simulink model "Model_simulink"  (R2015a)
settings: Solver=ode45  SolverMode=SingleTasking  StartTime=0.0  StopTime=20  RelTol=1e-3
values from neighbouring files (symbols this model uses):
  In = 130.7    [Skrypt_do_schematu.m]
  J = Js+Jmr    (= 5.82)    [Skrypt_do_schematu.m]
  Kp = 0.15*Un    (= 66)    [Skrypt_do_schematu.m]
  Kt = 10/(1.2*wn)    (= 0.0548810148593)    [Skrypt_do_schematu.m]
  Kw = J/(2*Kt*kz*Beta*psi)    [Skrypt_do_schematu.m]
  Lambda = 2    [Skrypt_do_schematu.m]
  m = T1    [Skrypt_do_schematu.m]
  Mn = psi * In    (= 350.156554572)    [Skrypt_do_schematu.m]
  psi = (Un-(Rt*In))/wn    (= 2.67908610996)    [Skrypt_do_schematu.m]
  Rt = 0.254    [Skrypt_do_schematu.m]
  T = Lt/Rt    (= 0.00641732283465)    [Skrypt_do_schematu.m]
  T1 = (B/2)*(1-sqrt(1-(4*T/B)))    [Skrypt_do_schematu.m]
  Un = 440    [Skrypt_do_schematu.m]
  Uz0 = (Lambda*In)*((Y*B1)/(B1-Beta))    [Skrypt_do_schematu.m]
  V = (Beta*(Y*Kp*B))/((B1-Beta)*Rt)    [Skrypt_do_schematu.m]
  wn = (2*pi*n)/60    (= 151.843644924)    [Skrypt_do_schematu.m]
  Y = 7.8/(2.5*In)    (= 0.0238714613619)    [Skrypt_do_schematu.m]
settings Model: Creator=user  LastModifiedBy=user
settings DataIOCC: SignalLoggingSaveFormat=ModelDataLogs
settings OptimizationCC: BlockReduction=off  BooleanDataType=off  ExpressionDepthLimit=2147483647
settings DebuggingCC: SaveWithParameterizedLinksMsg=none  UnderspecifiedInitializationDetection=Classic  MergeDetectMultiDrivingBlocksExec=none  SignalResolutionControl=TryResolveAllWithWarning  MultiTaskDSMMsg=warning  MultiTaskCondExecSysMsg=none  StateNameClashWarn=warning
settings HardwareCC: TargetUnknown=on

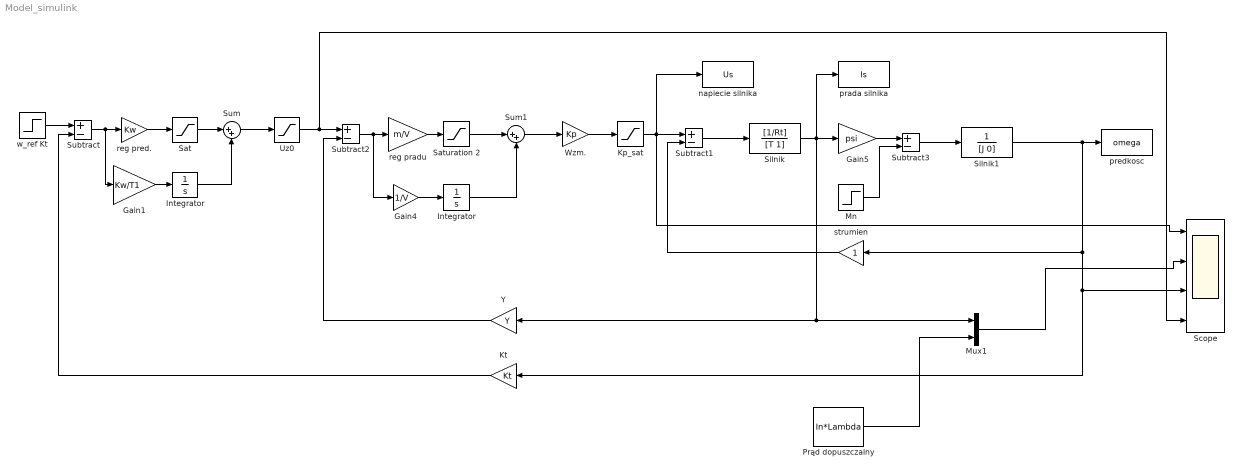
== system Model_simulink ==
  Gain1 : Gain  Gain=Kw/T1
  Gain4 : Gain  Gain=1/V
  Gain5 : Gain  Gain=psi
  Integrator : Integrator  LimitOutput=on  UpperSaturationLimit=10  LowerSaturationLimit=-10
  "Integrator " : Integrator  LimitOutput=on  UpperSaturationLimit=10  LowerSaturationLimit=-10
  Kp_sat : Saturate  UpperLimit=1.5*Un  LowerLimit=-1.5*Un
  Kt : Gain  Gain=Kt
  Mn : Step  After=Mn  SampleTime=0
  Mux1 : Mux  Inputs=2
  Prąd dopuszczalny : Constant  Value=In*Lambda
  Sat : Saturate  UpperLimit=10  LowerLimit=-10
  Saturation 2 : Saturate  UpperLimit=10  LowerLimit=-10
  Scope : Scope  NumInputPorts=4
      settings: YMin=-5~-5~-5~-5  YMax=5~5~5~5
  Silnik : TransferFcn  Numerator=[1/Rt]  Denominator=[T 1]
  Silnik1 : TransferFcn  Numerator=1  Denominator=[J 0]
  Subtract{,1..3} (4 alike) : Sum  Inputs=+-
  Sum : Sum  Inputs=|++
  Sum1 : Sum  Inputs=|++
  Uz0 : Saturate  UpperLimit=Uz0  LowerLimit=-Uz0
  Wzm. : Gain  Gain=Kp
  Y : Gain  Gain=Y
  napiecie silnika : ToWorkspace  VariableName=Us  SaveFormat=Timeseries  SampleTime=-1
  prada silnika : ToWorkspace  VariableName=Is  SaveFormat=Timeseries  SampleTime=-1
  predkosc : ToWorkspace  VariableName=omega  SaveFormat=Timeseries  SampleTime=-1
  reg pradu : Gain  Gain=m/V
  reg pred. : Gain  Gain=Kw
  strumien : Gain
  w_ref Kt : Step  Before=wn*Kt  After=wn*Kt  SampleTime=0
  wires:
  w_ref Kt/1 -> Subtract/1
  Subtract/1 -> Gain1/1, reg pred./1
  Gain1/1 -> Integrator/1
  Integrator/1 -> Sum/2
  Sum/1 -> Uz0/1
  Subtract2/1 -> Gain4/1, reg pradu/1
  reg pradu/1 -> Saturation 2/1
  Saturation 2/1 -> Sum1/1
  Sum1/1 -> Wzm./1
  Wzm./1 -> Kp_sat/1
  Gain4/1 -> "Integrator "/1
  "Integrator "/1 -> Sum1/2
  Subtract1/1 -> Silnik/1
  Silnik/1 -> prada silnika/1, Y/1, Mux1/1, Gain5/1
  Gain5/1 -> Subtract3/1
  Subtract3/1 -> Silnik1/1
  Mn/1 -> Subtract3/2
  strumien/1 -> Subtract1/2
  Kp_sat/1 -> Scope/1, napiecie silnika/1, Subtract1/1
  Y/1 -> Subtract2/2
  Mux1/1 -> Scope/2
  Prąd dopuszczalny/1 -> Mux1/2
  Uz0/1 -> Scope/4, Subtract2/1
  Silnik1/1 -> predkosc/1, strumien/1, Kt/1, Scope/3
  Kt/1 -> Subtract/2
  Sat/1 -> Sum/1
  reg pred./1 -> Sat/1
